simulink library "quat_inertial_estimate_mtv_lib"  (R2014b)
settings: Solver=ode45  StartTime=0.0  StopTime=10.0  RelTol=1e-3
libraries: util_quat_lib x4, util_info_lib x1, util_common_lib x1
settings Model: Creator=tgorton  LastModifiedBy=tgorton

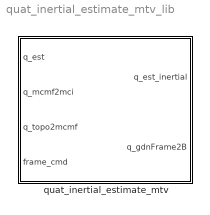
== system quat_inertial_estimate_mtv_lib ==
  quat_inertial_estimate_mtv : Subsystem
      mask Display:
      | color('blue')
      | text(0.05,0.02,'MoonEx',...
      |  	'HorizontalAlignment','Left',...
      | 	'VerticalAlignment','bottom')

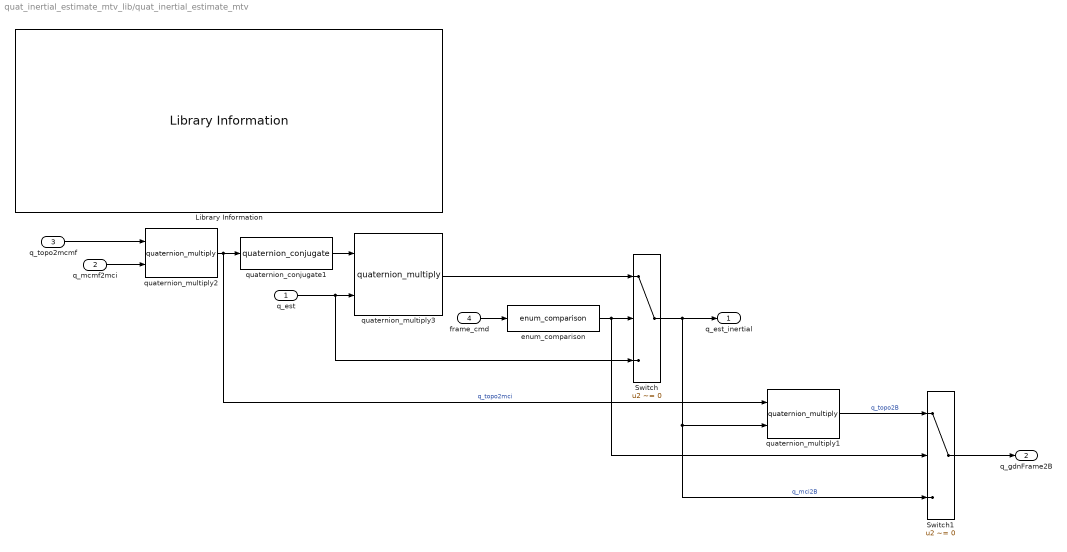
== system quat_inertial_estimate_mtv_lib/quat_inertial_estimate_mtv ==
  q_est : Inport
  q_mcmf2mci : Inport  Port=2
  q_topo2mcmf : Inport  Port=3
  frame_cmd : Inport  Port=4
  Library Information : util_info_lib/Library Information  owner='NONE'
  Switch : Switch  Criteria=u2 ~= 0
  Switch1 : Switch  Criteria=u2 ~= 0
  enum_comparison : util_common_lib/enum_comparison  comparison_type===
  quaternion_conjugate1 : util_quat_lib/quaternion_conjugate  SystemSampleTime=-1
  quaternion_multiply1 : util_quat_lib/quaternion_multiply  SystemSampleTime=-1
  quaternion_multiply2 : util_quat_lib/quaternion_multiply  SystemSampleTime=-1
  quaternion_multiply3 : util_quat_lib/quaternion_multiply  SystemSampleTime=-1
  q_est_inertial : Outport
  q_gdnFrame2B : Outport  Port=2
  wires:
  quaternion_multiply1/1 -> Switch1/1  "q_topo2B"
  Switch1/1 -> q_gdnFrame2B/1
  enum_comparison/1 -> Switch/2, Switch1/2
  q_topo2mcmf/1 -> quaternion_multiply2/1
  q_mcmf2mci/1 -> quaternion_multiply2/2
  quaternion_multiply2/1 -> quaternion_conjugate1/1, quaternion_multiply1/1  "q_topo2mci"
  quaternion_conjugate1/1 -> quaternion_multiply3/1
  frame_cmd/1 -> enum_comparison/1
  Switch/1 -> q_est_inertial/1, Switch1/3, quaternion_multiply1/2  "q_mci2B"
  quaternion_multiply3/1 -> Switch/1
  q_est/1 -> Switch/3, quaternion_multiply3/2
